simulink model "reaction_pendulum_LQR_KF"  (R2026a)
settings: Solver=FixedStepDiscrete  StopTime=inf  FixedStep=h  EnableMultiTasking=on
PreLoadFcn:
  | warning('off','MATLAB:dispatcher:InexactMatch');
InitFcn:
  | hwinit
undefined symbols (not defined in the file): A, B, C, Discrete, K, Time
libraries: ctrlSharedLib x1
settings Model: SimulationMode=external  ExtModeTrigDuration=100000  Creator=user  LastModifiedBy=jackh
settings DataIOCC: SignalLoggingSaveFormat=ModelDataLogs
settings DebuggingCC: UnderspecifiedInitializationDetection=Classic
settings HardwareCC: ProdHWDeviceType=32-bit Generic
settings RTWCC: SystemTargetFile=rtcon_rpend_usb2.tlc  TemplateMakefile=rtcon_rpend_vc_usb2_x64.tmf  Description=rpend RTDAC/USB2 (Visual C/C++)
settings STFCustomTargetCC: SystemTargetFile=rtcon_rpend_usb2.tlc  MultiwordLength=2048.0  ModelReferenceCompliant=off  CombineOutputUpdateFcns=on  MatFileLogging=on  GRTInterface=off  StartupMessage=on  Use_REALTIME_PRIORITY=off  Use_HIGH_PRIORITY=off
settings GRTTargetCC: ExtMode=on  ExtModeMexFile=rtcon_ext_comm  ModelReferenceCompliant=off  ParMdlRefBuildCompliant=off  CompOptLevelCompliant=off  ConcurrentExecutionCompliant=off  CPPClassGenCompliant=off

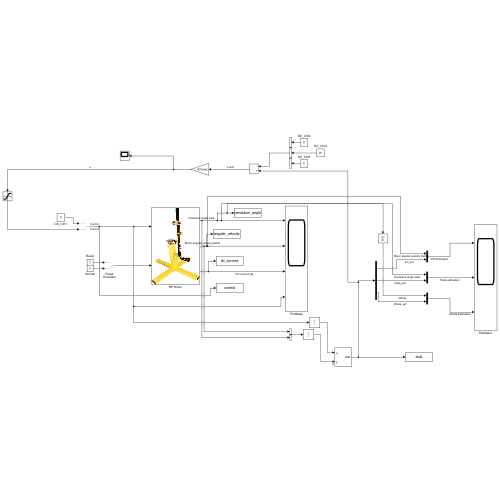
[thumbnail: Simulink's stored preview of the top-level diagram]
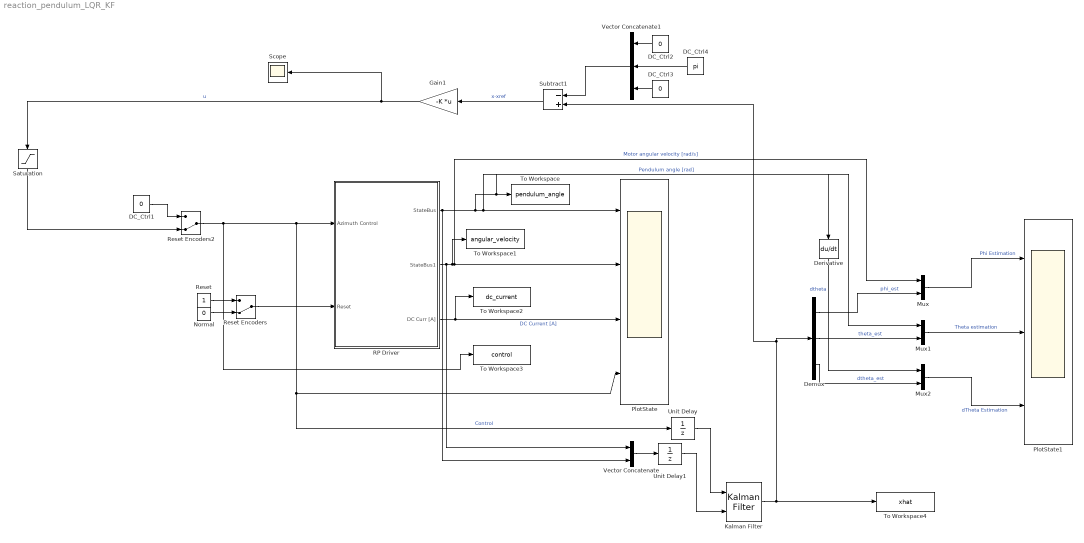
== system reaction_pendulum_LQR_KF ==
  DC_Ctrl1 : Constant  Value=0
  DC_Ctrl2 : Constant  Value=0
  DC_Ctrl3 : Constant  Value=0
  DC_Ctrl4 : Constant  Value=pi
  Demux : Demux  Outputs=3
  Derivative : Derivative
  Gain1 : Gain  Gain=-K  Multiplication=Matrix(K*u) (u vector)
  Kalman Filter : ctrlSharedLib/Kalman Filter  TimeDomain=Discrete-Time  UseCurrentEstimator=on  ModelSource=Individual A, B, C, D matrices  ModelSourceVariable=ss(0.95,1,1,0,1)  A=A  B=B  C=C  D=[0;0]  NumberOfStates=1  NumberOfInputs=1  NumberOfOutputs=1  Ts=0.01  InitialEstimateSource=Dialog  X0=0  P0=10  UseK=off  UseGH=off  G=1  TimeInvariantG=on  H=0  TimeInvariantH=on  NumberOfProcessNoiseInputs=1  Q=diag([0.1 0.1 0.001])  TimeInvariantQ=on  R=0.01  TimeInvariantR=on  N=0  TimeInvariantN=on  AddInputPort=on  AddEnablePort=off  OutputEstimatedY=off  OutputP=off
  Mux : Mux  Inputs=2
  Mux1 : Mux  Inputs=2
  Mux2 : Mux  Inputs=2
  Normal : Constant  Value=0
  PlotState : Scope  NumInputPorts=4
      settings: TimeSpan=40  ActiveDisplayYMinimum=2.69015  ActiveDisplayYMaximum=3.49754  DataLoggingMaxPoints=12000  DataLoggingVariableName=StateData
  PlotState1 : Scope  NumInputPorts=3
      settings: TimeSpan=40  ActiveDisplayYMinimum=-376.54923  ActiveDisplayYMaximum=79.51865  DataLoggingMaxPoints=12000  DataLoggingVariableName=ScopeData2
  RP Driver : Subsystem
      mask Display: image(imread('rwp.JPG'))
  Reset : Constant
  Reset Encoders : ManualSwitch  CurrentSetting=0
  Reset Encoders2 : ManualSwitch  CurrentSetting=0
  Saturation : Saturate  UpperLimit=1  LowerLimit=-1
  Scope : Scope
      settings: ActiveDisplayYMinimum=-0.61302  ActiveDisplayYMaximum=2.35708
  Subtract1 : Sum  Inputs=-+
  To Workspace : ToWorkspace  VariableName=pendulum_angle  SaveFormat=Timeseries  SampleTime=-1
  To Workspace1 : ToWorkspace  VariableName=angular_velocity  SaveFormat=Timeseries  SampleTime=-1
  To Workspace2 : ToWorkspace  VariableName=dc_current  SaveFormat=Timeseries  SampleTime=-1
  To Workspace3 : ToWorkspace  VariableName=control  SaveFormat=Timeseries  SampleTime=-1
  To Workspace4 : ToWorkspace  VariableName=xhat  SaveFormat=Timeseries  SampleTime=-1
  Unit Delay : UnitDelay  SampleTime=0.01
  Unit Delay1 : UnitDelay  SampleTime=0.01
  Vector Concatenate : Concatenate
  Vector Concatenate1 : Concatenate  NumInputs=3
  wires:
  Normal/1 -> Reset Encoders/2
  Reset/1 -> Reset Encoders/1
  Reset Encoders/1 -> RP Driver/2(Reset)
  RP Driver/3(DC Curr [A]) -> To Workspace2/1, PlotState/3  "DC Current [A]"
  Reset Encoders2/1 -> Unit Delay/1, PlotState/4, RP Driver/1(Azimuth Control), To Workspace3/1  "Control"
  RP Driver/2(StateBus1) -> Mux/1, PlotState/2, To Workspace1/1, Vector Concatenate/1  "Motor angular velocity [rad/s]"
  RP Driver/1(StateBus) -> Mux1/1, PlotState/1, Derivative/1, To Workspace/1, Vector Concatenate/2  "Pendulum angle [rad]"
  Vector Concatenate/1 -> Unit Delay1/1
  Unit Delay1/1 -> Kalman Filter/2
  Demux/3 -> Mux2/2  "dtheta_est"
  Demux/2 -> Mux1/2  "theta_est"
  Demux/1 -> Mux/2  "phi_est"
  Derivative/1 -> Mux2/1  "dtheta"
  Mux/1 -> PlotState1/1  "Phi Estimation"
  Mux1/1 -> PlotState1/2  "Theta estimation"
  Mux2/1 -> PlotState1/3  "dTheta Estimation"
  DC_Ctrl2/1 -> Vector Concatenate1/1
  DC_Ctrl3/1 -> Vector Concatenate1/3
  DC_Ctrl4/1 -> Vector Concatenate1/2
  Gain1/1 -> Scope/1, Saturation/1  "u"
  Saturation/1 -> Reset Encoders2/2
  DC_Ctrl1/1 -> Reset Encoders2/1
  Unit Delay/1 -> Kalman Filter/1
  Kalman Filter/1 -> To Workspace4/1, Demux/1, Subtract1/2
  Vector Concatenate1/1 -> Subtract1/1
  Subtract1/1 -> Gain1/1  "x-xref"

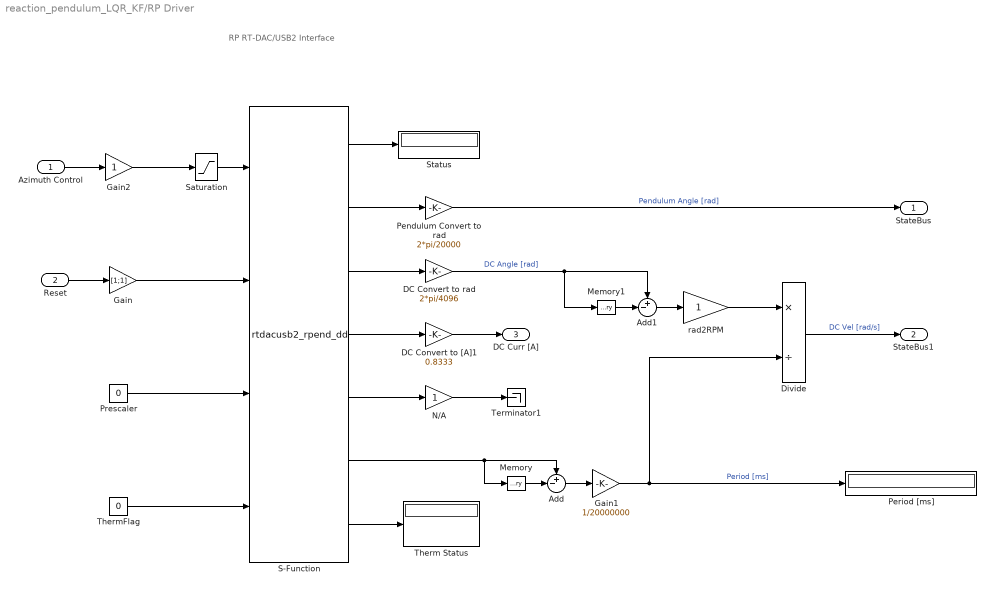
== system reaction_pendulum_LQR_KF/RP Driver ==
  note: RP RT-DAC/USB2
      | Interface
  Azimuth Control : Inport
  Reset : Inport  Port=2
  Add : Sum  Inputs=+-|
  Add1 : Sum  Inputs=+-|
  DC Convert to [A]1 : Gain  Gain=0.8333  SaturateOnIntegerOverflow=on  OutDataTypeStr=Inherit: Same as input  ParamDataTypeStr=Inherit: Same as input
  DC Convert to rad : Gain  Gain=2*pi/4096  SaturateOnIntegerOverflow=on  OutDataTypeStr=Inherit: Same as input  ParamDataTypeStr=Inherit: Same as input
  Divide : Product  Inputs=*/
  Gain : Gain  Gain=[1;1]
  Gain1 : Gain  Gain=1/20000000
  Gain2 : Gain
  Memory : Memory
  Memory1 : Memory
  N/A : Gain  SaturateOnIntegerOverflow=on  OutDataTypeStr=Inherit: Same as input  ParamDataTypeStr=Inherit: Same as input
  Pendulum Convert to rad : Gain  Gain=2*pi/20000  SaturateOnIntegerOverflow=on  OutDataTypeStr=Inherit: Same as input  ParamDataTypeStr=Inherit: Same as input
  Period [ms] : Display
  Prescaler : Constant  Value=0
  S-Function : S-Function  FunctionName=rtdacusb2_rpend_dd  Parameters=1, h  SFunctionDeploymentMode=off  EnableBusSupport=off
  Saturation : Saturate  UpperLimit=1  LowerLimit=-1
  Status : Display
  Terminator1 : Terminator
  Therm Status : Display
  ThermFlag : Constant  Value=0
  rad2RPM : Gain  SaturateOnIntegerOverflow=on  OutDataTypeStr=Inherit: Same as input  ParamDataTypeStr=Inherit: Same as input
  StateBus : Outport  VectorParamsAs1DForOutWhenUnconnected=off
  StateBus1 : Outport  Port=2  VectorParamsAs1DForOutWhenUnconnected=off
  DC Curr [A] : Outport  Port=3  VectorParamsAs1DForOutWhenUnconnected=off
  wires:
  S-Function/7 -> Therm Status/1
  S-Function/5 -> N/A/1
  S-Function/4 -> DC Convert to [A]1/1
  ThermFlag/1 -> S-Function/4
  Prescaler/1 -> S-Function/3
  Gain/1 -> S-Function/2
  DC Convert to [A]1/1 -> DC Curr [A]/1
  Divide/1 -> StateBus1/1  "DC Vel [rad/s]"
  rad2RPM/1 -> Divide/1
  Add1/1 -> rad2RPM/1
  Memory1/1 -> Add1/2
  N/A/1 -> Terminator1/1
  S-Function/6 -> Add/1, Memory/1
  Gain2/1 -> Saturation/1
  Gain1/1 -> Period [ms]/1, Divide/2  "Period [ms]"
  Add/1 -> Gain1/1
  Memory/1 -> Add/2
  DC Convert to rad/1 -> Add1/1, Memory1/1  "DC Angle [rad]"
  S-Function/3 -> DC Convert to rad/1
  Pendulum Convert to rad/1 -> StateBus/1  "Pendulum Angle [rad]"
  S-Function/2 -> Pendulum Convert to rad/1
  S-Function/1 -> Status/1
  Saturation/1 -> S-Function/1
  Reset/1 -> Gain/1
  Azimuth Control/1 -> Gain2/1
